simulink library "CF3"  (R2013b)
settings: Solver=ode45  StartTime=0.0  StopTime=10.0  RelTol=1e-3
settings Model: Creator=Nam  LastModifiedBy=Nam

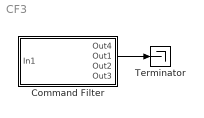
== system CF3 ==
  Command Filter : Subsystem  mask{Integrator1_init=0, omega_n1=2*pi*1, omega_n2=2*pi*1, zeta=.9}
      mask init:
      | zeta > 0
      | zeta <= 1
      mask DialogControl Control3_copy_copy Prompt: Initial value Integrator1
      mask DialogControl Control4 Prompt: omega_n1
      mask DialogControl Control5 Prompt: omega_n2
      mask DialogControl Control6 Prompt: zeta
  Terminator : Terminator
  wires:
  Command Filter/2(Out1) -> Terminator/1

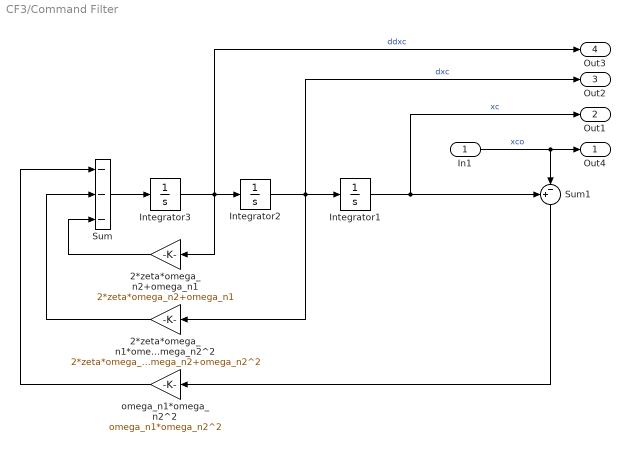
== system CF3/Command Filter ==
  In1 : Inport
  2*zeta*omega_n1*omega_n2+omega_n2^2 : Gain  Gain=2*zeta*omega_n1*omega_n2+omega_n2^2
  2*zeta*omega_n2+omega_n1 : Gain  Gain=2*zeta*omega_n2+omega_n1
  Integrator1 : Integrator  InitialCondition=Integrator1_init
  Integrator2 : Integrator
  Integrator3 : Integrator
  Sum : Sum  Inputs=---
  Sum1 : Sum  Inputs=+-|
  omega_n1*omega_n2^2 : Gain  Gain=omega_n1*omega_n2^2
  Out4 : Outport
  Out1 : Outport  Port=2
  Out2 : Outport  Port=3
  Out3 : Outport  Port=4
  wires:
  Integrator3/1 -> 2*zeta*omega_n2+omega_n1/1, Out3/1, Integrator2/1  "ddxc"
  In1/1 -> Out4/1, Sum1/2  "xco"
  Integrator2/1 -> 2*zeta*omega_n1*omega_n2+omega_n2^2/1, Out2/1, Integrator1/1  "dxc"
  Sum1/1 -> omega_n1*omega_n2^2/1
  Integrator1/1 -> Out1/1, Sum1/1  "xc"
  2*zeta*omega_n2+omega_n1/1 -> Sum/3
  Sum/1 -> Integrator3/1
  omega_n1*omega_n2^2/1 -> Sum/1
  2*zeta*omega_n1*omega_n2+omega_n2^2/1 -> Sum/2
